simulink model "turkpupr"  (R2023a)
settings: Solver=ode45  StartTime=0.0  StopTime=5  FixedStep=0.0001  RelTol=1e-8  EnableMultiTasking=on
settings Model: Creator=Пользователь  LastModifiedBy=k.balkunov
settings SolverCC: AlgebraicLoopSolver=TrustRegion
settings DataIOCC: LimitDataPoints=on  SaveFormat=Array  ReturnWorkspaceOutputs=off
settings OptimizationCC: ExpressionDepthLimit=2147483647  LifeSpan=inf
settings DebuggingCC: UnderspecifiedInitializationDetection=Classic  MergeDetectMultiDrivingBlocksExec=none  SolverPrmCheckMsg=warning  UnconnectedInputMsg=warning  UnconnectedOutputMsg=warning  UnconnectedLineMsg=warning  StateNameClashWarn=warning  SFUnexpectedBacktrackingDiag=warning  SFNoUnconditionalDefaultTransitionDiag=warning  SFExecutionAtInitializationDiag=none  ArithmeticOperatorsInVariantConditions=warning
settings HardwareCC: ProdBitPerPointer=32  ProdBitPerSizeT=32  ProdBitPerPtrDiffT=32  ProdLargestAtomicFloat=None  ProdIntDivRoundTo=Undefined  ProdEndianess=Unspecified  ProdWordSize=32  ProdHWDeviceType=32-bit Generic
settings ModelReferenceCC: EnableRefExpFcnMdlSchedulingChecks=on  PropagateSignalLabelsOutOfModel=off
settings SFSimCC: SimUseLocalCustomCode=off  CustomCodeUndefinedFunction=UseInterfaceOnly
settings RTWCC: RTWUseLocalCustomCode=off
settings CodeAppCC: StateflowObjectComments=on
settings GRTTargetCC: TargetLangStandard=C89/C90 (ANSI)
settings ConfigComp: CovMetricSettings=dw  CovSaveCumulativeToWorkspaceVar=on  CovSaveSingleToWorkspaceVar=on  CovExternalEMLEnable=off

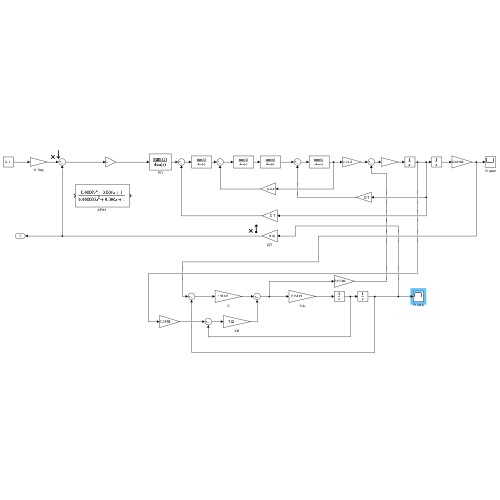
[thumbnail: Simulink's stored preview of the top-level diagram]
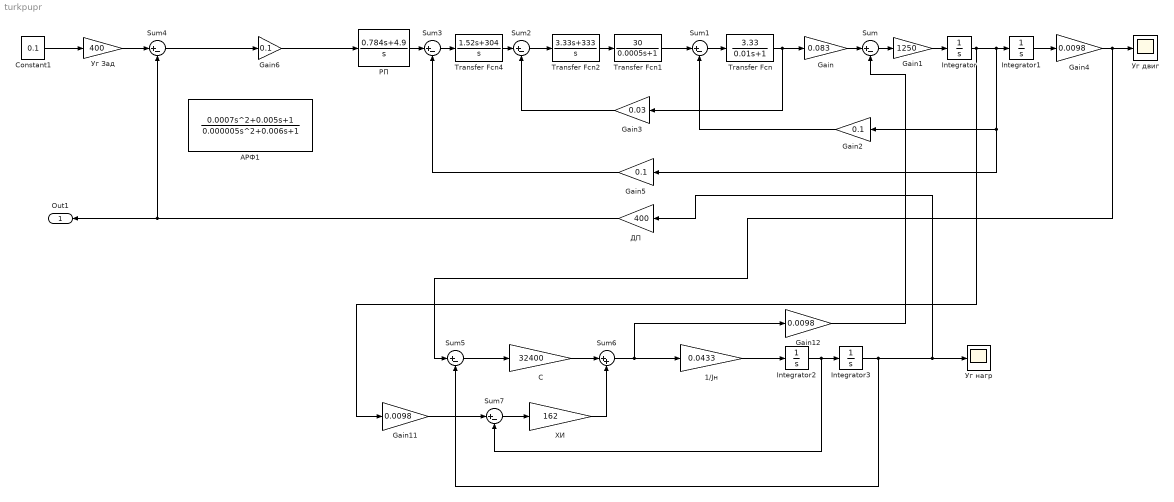
== system turkpupr ==
  1/Jн : Gain  Gain=0.0433
  Constant1 : Constant  Value=0.1
  Gain : Gain  Gain=0.083
  Gain1 : Gain  Gain=1250
  Gain11 : Gain  Gain=0.0098
  Gain12 : Gain  Gain=0.0098
  Gain2 : Gain  Gain=0.1
  Gain3 : Gain  Gain=0.03
  Gain4 : Gain  Gain=0.0098
  Gain5 : Gain  Gain=0.1
  Gain6 : Gain  Gain=0.1
  Integrator{,1..3} (4 alike) : Integrator
  Sum{,1..5,7} (7 alike) : Sum  Inputs=|+-
  Sum6 : Sum  Inputs=|++
  Transfer Fcn : TransferFcn  Numerator=[3.33]  Denominator=[0.01 1]
  Transfer Fcn1 : TransferFcn  Numerator=[30]  Denominator=[0.0005 1]
  Transfer Fcn2 : TransferFcn  Numerator=[3.33 333]  Denominator=[1 0]
  Transfer Fcn4 : TransferFcn  Numerator=[1.52 304]  Denominator=[1 0]
  "АРФ1 " : TransferFcn  Numerator=[0.0007 0.005 1]  Denominator=[0.000005 0.006 1]
  ДП : Gain  Gain=400
  РП : TransferFcn  Numerator=[0.784 4.9]  Denominator=[1 0]
  С : Gain  Gain=32400
  Уг Зад : Gain  Gain=400
  Уг двиг : Scope
  Уг нагр : Scope
  ХИ : Gain  Gain=162
  Out1 : Outport
  wires:
  Sum1/1 -> Transfer Fcn/1
  Gain/1 -> Sum/1
  Sum/1 -> Gain1/1
  Gain1/1 -> Integrator/1
  Integrator/1 -> Gain11/1, Integrator1/1, Gain5/1, Gain2/1
  Transfer Fcn1/1 -> Sum1/1
  Sum2/1 -> Transfer Fcn2/1
  Transfer Fcn/1 -> Gain3/1, Gain/1
  Gain2/1 -> Sum1/2
  Transfer Fcn2/1 -> Transfer Fcn1/1
  Sum3/1 -> Transfer Fcn4/1
  Transfer Fcn4/1 -> Sum2/1
  Gain3/1 -> Sum2/2
  Gain5/1 -> Sum3/2
  Integrator1/1 -> Gain4/1
  Gain4/1 -> Sum5/1, Уг двиг/1
  ДП/1 -> Out1/1, Sum4/2
  Уг Зад/1 -> Sum4/1
  Constant1/1 -> Уг Зад/1
  Sum5/1 -> С/1
  С/1 -> Sum6/1
  1/Jн/1 -> Integrator2/1
  Integrator2/1 -> Sum7/2, Integrator3/1
  Sum6/1 -> Gain12/1, 1/Jн/1
  Integrator3/1 -> ДП/1, Уг нагр/1, Sum5/2
  Sum7/1 -> ХИ/1
  Gain11/1 -> Sum7/1
  ХИ/1 -> Sum6/2
  Gain12/1 -> Sum/2
  Sum4/1 -> Gain6/1
  Gain6/1 -> РП/1
  РП/1 -> Sum3/1
